simulink model "NE_Red_Rooster_Delta_B_28may"  (R2019b)
settings: Solver=FixedStepAuto  StartTime=0.0  StopTime=inf  FixedStep=0.0005  RelTol=1e-3
PreLoadFcn:
  | waijung.modelPreload; % Required for working with Waijung Blockset. Do not remove.
undefined symbols (not defined in the file): ARM, DiscIntNeverNeededParam, HSEOSC, Link, LQFP100, MDK, ST, STM32F407VG
libraries: simulink x30, stm32f4_i2c_lib x22, stm32f4_io_lib x6, stm32f4_reset_lib x1, stm32f4_device_config_lib x1
(part 2 of 5)

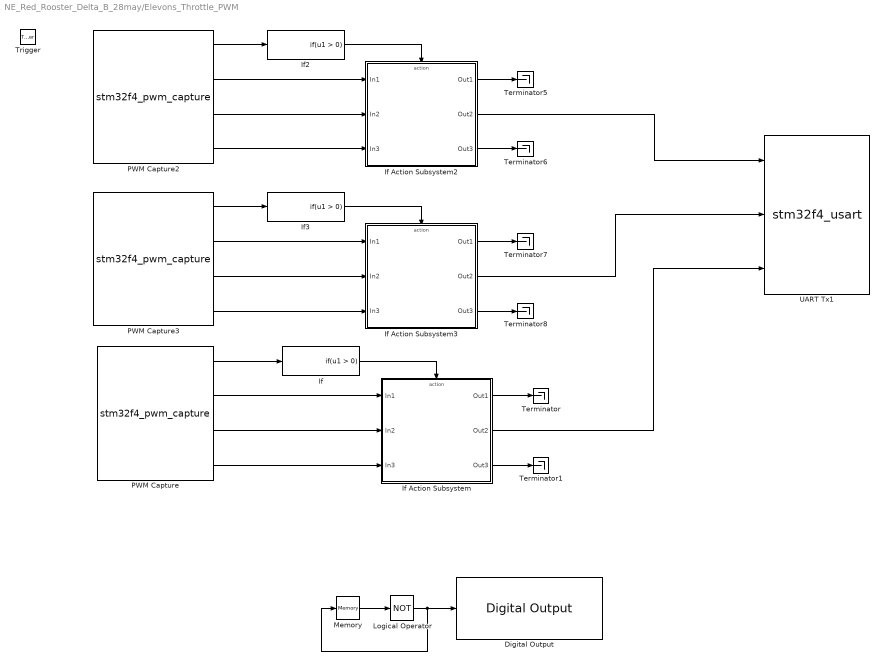
== system NE_Red_Rooster_Delta_B_28may/Elevons_Throttle_PWM ==
  Trigger : TriggerPort  VariantControl=Variant
  Digital Output : stm32f4_io_lib/Digital Output  use_bitband=on  port=D  speed=100  porttype=Push Pull  porttypestr=PP  use_pin0=off  use_pin1=off  use_pin2=off  use_pin3=off  use_pin4=off  use_pin5=off  use_pin6=off  use_pin7=off  use_pin8=off  use_pin9=off  use_pin10=off  use_pin11=off  use_pin12=on  use_pin13=off  use_pin14=off  use_pin15=off  pinstr=GPIO_Pin_12  usedpinarray="[0  0  0  0  0  0  0  0  0  0  0  0  1  0  0  0]"  bitbandingstr="#define Elevons_Throttle_PWMDigitalOutput_D12 Peripheral_BB(GPIOD->ODR, 12)  /* Output pin */"  sampletime=-1  sampletimestr=-1  blockid=Elevons_Throttle_PWMDigitalOutput  enablecustomportlabel=off  globalinit=off  cinputportlabel=In1, In2  coutputportlabel=0
  If : If  ShowElse=off
  If Action Subsystem : Subsystem  TreatAsAtomicUnit=on
  If Action Subsystem2 : Subsystem  TreatAsAtomicUnit=on
  If Action Subsystem3 : Subsystem  TreatAsAtomicUnit=on
  If2 : If  ShowElse=off
  If3 : If  ShowElse=off
  Logical Operator : Logic  Operator=NOT  AllPortsSameDT=off  OutDataTypeStr=boolean
  Memory : Memory  InheritSampleTime=on
  PWM Capture : S-Function  FunctionName=stm32f4_pwm_capture  Parameters=conf,inputporttype,inputportwidth,outputporttype,outputportwidth,optionstring,sampletime,blockid  SFunctionDeploymentMode=off  EnableBusSupport=off  mask(stm32f4_pwm_capture){conf=Capture, timer=8, lasttimer=8, pin=C6, pintype=Pull Up, edge=Rising, datatype=single, portpinstr=0, sampletime=-1, blockid=Elevons_Throttle_PWMPWMCapture, inputporttype=[], inputportwidth=[], inputportlabel={}, outputporttype=[3 1 1 1], outputportwidth=[], outputportlabel={'READY','+Width (sec)','+Duty (%)','Frequency (Hz)'}, compat=0, optionstring=["8","2","C","6","1","16","Rising","UP","float"]}
      mask prompts: conf "Configuration"; lasttimer "Last Timer"; pin "Capture Pin"; pintype "Capture Pin Type (Pull-Up/Pull-Down)"; edge "Capture Edge"; datatype "Output data type"; portpinstr "Port Pin String"; sampletime "Sample time (sec)"; blockid "Block ID"; inputporttype "Input Port Type"; inputportwidth "Input Port Width"; inputportlabel "Input Port Label"; outputporttype "Output Port Type"; outputportwidth "Output Port Width"; outputportlabel "Output port label"; compat "Compatibility (Reserved for future use)"; optionstring "String(s) to be passed to TLC"
      mask help:
      | Capture Edge:
      |  Rising - PWM period start from rising edge of pulse N to rising edge of pulse N+1
      |  Falling - PWM period start from falling edge of pulse N to falling edge of pulse N+1
      | Capture data type:
      |  Capture data type, selectable to double or single.
      |
      | Output:
      |  READY - indicate the status of capture, a non-zero value indicate data is ready.
      |  +Width - positive pulse width, in unit of second.
      |  +Duty - positive duty cycle, 0 to 100%
      |  Frequency - signal frequency in unit of Hz
      |
      | Note: caprure period should not longer than 1 second (Maximum limit is 3 seconds)
      mask init:
      | stm32f4_pwm_capture_callback('init');
      mask Help: web(fullfile(waijungdocroot,'stm32f4_pwm_capture.htm'), '-browser')
      mask TypeOptions conf: Capture
      mask Callback conf: stm32f4_pwm_capture_callback('conf');
      mask TypeOptions timer: 1 | 2 | 3 | 4 | 5 | 8
      mask Callback timer: stm32f4_pwm_capture_callback('timer');
      mask TypeOptions pin: Not used | C6 | C7 | C8 | C9
      mask TypeOptions pintype: None | Pull Up | Pull Down
      mask TypeOptions edge: Rising | Falling
      mask TypeOptions datatype: double | single
      mask Callback sampletime: stm32f4_pwm_capture_callback('sampletime');
      mask Callback blockid: stm32f4_pwm_capture_callback('blockid');
      mask Display: text(0.05, 0.5, 'Timer: 8 (16 bit)\nInput Pin: C6\nEdge: Rising\nTs (sec): -1','ver','middle','hor','left'); port_label('output', 1,'READY'); port_label('output', 2,'+Width (sec)'); port_label('output', 3,'+Duty (%)'); port_label('output', 4,'Frequency (Hz)');
  PWM Capture2 : S-Function  FunctionName=stm32f4_pwm_capture  Parameters=conf,inputporttype,inputportwidth,outputporttype,outputportwidth,optionstring,sampletime,blockid  SFunctionDeploymentMode=off  EnableBusSupport=off  mask(stm32f4_pwm_capture){conf=Capture, timer=1, lasttimer=1, pin=E9, pintype=Pull Up, edge=Rising, datatype=single, portpinstr=0, sampletime=-1, blockid=Elevons_Throttle_PWMPWMCapture2, inputporttype=[], inputportwidth=[], inputportlabel={}, outputporttype=[3 1 1 1], outputportwidth=[], outputportlabel={'READY','+Width (sec)','+Duty (%)','Frequency (Hz)'}, compat=0, optionstring=["1","2","E","9","1","16","Rising","UP","float"]}
      mask prompts: conf "Configuration"; lasttimer "Last Timer"; pin "Capture Pin"; pintype "Capture Pin Type (Pull-Up/Pull-Down)"; edge "Capture Edge"; datatype "Output data type"; portpinstr "Port Pin String"; sampletime "Sample time (sec)"; blockid "Block ID"; inputporttype "Input Port Type"; inputportwidth "Input Port Width"; inputportlabel "Input Port Label"; outputporttype "Output Port Type"; outputportwidth "Output Port Width"; outputportlabel "Output port label"; compat "Compatibility (Reserved for future use)"; optionstring "String(s) to be passed to TLC"
      mask help:
      | Capture Edge:
      |  Rising - PWM period start from rising edge of pulse N to rising edge of pulse N+1
      |  Falling - PWM period start from falling edge of pulse N to falling edge of pulse N+1
      | Capture data type:
      |  Capture data type, selectable to double or single.
      |
      | Output:
      |  READY - indicate the status of capture, a non-zero value indicate data is ready.
      |  +Width - positive pulse width, in unit of second.
      |  +Duty - positive duty cycle, 0 to 100%
      |  Frequency - signal frequency in unit of Hz
      |
      | Note: caprure period should not longer than 1 second (Maximum limit is 3 seconds)
      mask init:
      | stm32f4_pwm_capture_callback('init');
      mask Help: web(fullfile(waijungdocroot,'stm32f4_pwm_capture.htm'), '-browser')
      mask TypeOptions conf: Capture
      mask Callback conf: stm32f4_pwm_capture_callback('conf');
      mask TypeOptions timer: 1 | 2 | 3 | 4 | 5 | 8
      mask Callback timer: stm32f4_pwm_capture_callback('timer');
      mask TypeOptions pin: Not used | A8 | E9 | A9 | E11 | A10 | E13 | A11 | E14
      mask TypeOptions pintype: None | Pull Up | Pull Down
      mask TypeOptions edge: Rising | Falling
      mask TypeOptions datatype: double | single
      mask Callback sampletime: stm32f4_pwm_capture_callback('sampletime');
      mask Callback blockid: stm32f4_pwm_capture_callback('blockid');
      mask Display: text(0.05, 0.5, 'Timer: 1 (16 bit)\nInput Pin: E9\nEdge: Rising\nTs (sec): -1','ver','middle','hor','left'); port_label('output', 1,'READY'); port_label('output', 2,'+Width (sec)'); port_label('output', 3,'+Duty (%)'); port_label('output', 4,'Frequency (Hz)');
  PWM Capture3 : S-Function  FunctionName=stm32f4_pwm_capture  Parameters=conf,inputporttype,inputportwidth,outputporttype,outputportwidth,optionstring,sampletime,blockid  SFunctionDeploymentMode=off  EnableBusSupport=off  mask(stm32f4_pwm_capture){conf=Capture, timer=3, lasttimer=3, pin=C7, pintype=Pull Up, edge=Rising, datatype=single, portpinstr=0, sampletime=-1, blockid=Elevons_Throttle_PWMPWMCapture3, inputporttype=[], inputportwidth=[], inputportlabel={}, outputporttype=[3 1 1 1], outputportwidth=[], outputportlabel={'READY','+Width (sec)','+Duty (%)','Frequency (Hz)'}, compat=0, optionstring=["3","1","C","7","2","16","Rising","UP","float"]}
      mask prompts: conf "Configuration"; lasttimer "Last Timer"; pin "Capture Pin"; pintype "Capture Pin Type (Pull-Up/Pull-Down)"; edge "Capture Edge"; datatype "Output data type"; portpinstr "Port Pin String"; sampletime "Sample time (sec)"; blockid "Block ID"; inputporttype "Input Port Type"; inputportwidth "Input Port Width"; inputportlabel "Input Port Label"; outputporttype "Output Port Type"; outputportwidth "Output Port Width"; outputportlabel "Output port label"; compat "Compatibility (Reserved for future use)"; optionstring "String(s) to be passed to TLC"
      mask help:
      | Capture Edge:
      |  Rising - PWM period start from rising edge of pulse N to rising edge of pulse N+1
      |  Falling - PWM period start from falling edge of pulse N to falling edge of pulse N+1
      | Capture data type:
      |  Capture data type, selectable to double or single.
      |
      | Output:
      |  READY - indicate the status of capture, a non-zero value indicate data is ready.
      |  +Width - positive pulse width, in unit of second.
      |  +Duty - positive duty cycle, 0 to 100%
      |  Frequency - signal frequency in unit of Hz
      |
      | Note: caprure period should not longer than 1 second (Maximum limit is 3 seconds)
      mask init:
      | stm32f4_pwm_capture_callback('init');
      mask Help: web(fullfile(waijungdocroot,'stm32f4_pwm_capture.htm'), '-browser')
      mask TypeOptions conf: Capture
      mask Callback conf: stm32f4_pwm_capture_callback('conf');
      mask TypeOptions timer: 1 | 2 | 3 | 4 | 5 | 8
      mask Callback timer: stm32f4_pwm_capture_callback('timer');
      mask TypeOptions pin: Not used | A6 | B4 | C6 | A7 | B5 | C7 | B0 | C8 | B1 | C9
      mask TypeOptions pintype: None | Pull Up | Pull Down
      mask TypeOptions edge: Rising | Falling
      mask TypeOptions datatype: double | single
      mask Callback sampletime: stm32f4_pwm_capture_callback('sampletime');
      mask Callback blockid: stm32f4_pwm_capture_callback('blockid');
      mask Display: text(0.05, 0.5, 'Timer: 3 (16 bit)\nInput Pin: C7\nEdge: Rising\nTs (sec): -1','ver','middle','hor','left'); port_label('output', 1,'READY'); port_label('output', 2,'+Width (sec)'); port_label('output', 3,'+Duty (%)'); port_label('output', 4,'Frequency (Hz)');
  Terminator{,1,5..8} (6 alike) : Terminator
  UART Tx1 : S-Function  Priority=1  FunctionName=stm32f4_usart  Parameters=configuration,uartmodule,transfer,baudrate,inputtype,outputtype,confstr,binheaderarray,binterminatorarray,asciiheader,asciiterminator,bindatalength,packetmode,varname,sampletime,sampletimestr,blockid  SFunctionDeploymentMode=off  EnableBusSupport=off  mask(stm32f4_usart){configuration=Tx, uartmodule=2, baudrate=115200, databits=8, parity=No, stopbit=1, remaptxpin=Not used, remaprxpin=Not used, flowcontrol=None, remapctspin=Not used, remaprtspin=Not used, advanceoptions=off, rxbuffersize=512, txbuffersize=512, transfer=Blocking, packetmode=Binary, binheader='45', binterminator='2E', porttype_double=0, porttype_single=3, porttype_int8=0, porttype_uint8=0, porttype_int16=0, porttype_uint16=0, porttype_int32=0, porttype_uint32=0, asciiformat='%f, %f', rx_asciiterminator=CRLF (0x0D 0x0A - "\r\n"), tx_asciiterminator=CRLF (0x0D 0x0A - "\r\n"), storagename=<empty>, varname=, inputtype=[3  1 1 1], outputtype=[0], binheaderarray=[1 69], binterminatorarray=[1 46], bindatalength=12, asciiheader='%f, %f\r\n', asciiterminator=[2 13 10], sampletime=-1, sampletimestr=-1, blockid=Elevons_Throttle_PWMUARTTx1, confstr=[ "dummy", "0", "*", "*", "0", "*", "*", "0", "*", "*", "0", "*", "*", "1", "4", "6", "1", "4", "5", "512", "512", "1", "2", "115200", "8", "No", "1", "None", "USART2"], lastmodule=1}
      mask prompts: uartmodule "UART Module"; baudrate "Baud rate (bps)"; databits "Data bits"; stopbit "Stop bit"; remaptxpin "Tx Pin"; remaprxpin "Rx Pin"; flowcontrol "Hardware flow control"; remapctspin "HW Flow control, CTS Pin"; remaprtspin "HW Flow control, RTS Pin"; advanceoptions "Advance options"; rxbuffersize "Rx buffer size (bytes)"; txbuffersize "Tx buffer size (bytes)"; packetmode "Packet mode"; binheader "Binary header (example: '7E 7E')"; binterminator "Binary terminator (example: '03 03')"; porttype_double "Number of data port, type DOUBLE"; porttype_single "Number of data port, type SINGLE"; porttype_int8 "Number of data port, type INT8"; porttype_uint8 "Number of data port, type UINT8"; porttype_int16 "Number of data port, type INT16"; porttype_uint16 "Number of data port, type UINT16"; porttype_int32 "Number of data port, type INT32"; porttype_uint32 "Number of data port, type UINT32"; asciiformat "Ascii format"; rx_asciiterminator "End of packet"; tx_asciiterminator "End of packet"; storagename "Buffer"; varname "Var name"; inputtype "Input data type"; outputtype "Output data type"; binheaderarray "Binary header"; binterminatorarray "Binary terminator"; bindatalength "Binary data length"; asciiheader "Ascii header (printf format)"; asciiterminator "Ascii terminator"; sampletime "Sample time (sec)"; sampletimestr "Compiled sample time (sec) in string"; confstr "Configuration string"; lastmodule "Last module selected"
      mask help:
      | Data type for Ascii format
      | %u, %i, %d, %o, %x: uint32
      | %e, %g, %f: single
      | %c: int8
      mask init:
      | stm32f4_usart_callback('init');
      mask Help: web(fullfile(waijungdocroot,'stm32f4_usart_tx.htm'), '-browser')
      mask TypeOptions configuration: Setup | Tx | Rx
      mask Callback configuration: stm32f4_usart_callback('configuration');
      mask TypeOptions uartmodule: 1 | 2 | 3 | 4 | 5 | 6
      mask Callback uartmodule: stm32f4_usart_callback('uartmodule');
      mask Callback baudrate: stm32f4_usart_callback('baudrate');
      mask TypeOptions databits: 8
      mask TypeOptions parity: No | Odd | Even
      mask TypeOptions stopbit: 0.5 | 1 | 1.5 | 2
      mask TypeOptions remaptxpin: Not used | A9 | B6
      mask TypeOptions remaprxpin: Not used | A10 | B7
      mask TypeOptions flowcontrol: None | RTS | CTS | RTS/CTS
      mask Callback flowcontrol: stm32f4_usart_callback('flowcontrol');
      mask TypeOptions remapctspin: Not used | A11
      mask TypeOptions remaprtspin: Not used | A12
      mask Callback advanceoptions: stm32f4_usart_callback('advanceoptions');
      mask TypeOptions rxbuffersize: 16 | 32 | 64 | 128 | 256 | 512 | 1024 | 2048
      mask TypeOptions txbuffersize: 16 | 32 | 64 | 128 | 256 | 512 | 1024 | 2048
      mask TypeOptions transfer: Blocking | Non-Blocking
      mask Callback transfer: stm32f4_usart_callback('transfer');
      mask TypeOptions packetmode: Ascii | Binary | Binary Vector | String Buffer | Raw Buffer
      mask Callback packetmode: stm32f4_usart_callback('packetmode');
      mask Callback binheader: stm32f4_usart_callback('binheader');
      mask Callback binterminator: stm32f4_usart_callback('binterminator');
      mask Callback porttype_double: stm32f4_usart_callback('porttype');
      mask Callback porttype_single: stm32f4_usart_callback('porttype');
      mask Callback porttype_int8: stm32f4_usart_callback('porttype');
      mask Callback porttype_uint8: stm32f4_usart_callback('porttype');
      mask Callback porttype_int16: stm32f4_usart_callback('porttype');
      mask Callback porttype_uint16: stm32f4_usart_callback('porttype');
      mask Callback porttype_int32: stm32f4_usart_callback('porttype');
      mask Callback porttype_uint32: stm32f4_usart_callback('porttype');
      mask Callback asciiformat: stm32f4_usart_callback('asciiformat');
      mask TypeOptions rx_asciiterminator: CR (0x0D - "\r") | LF (0x0A - "\n") | CRLF (0x0D 0x0A - "\r\n")
      mask Callback rx_asciiterminator: stm32f4_usart_callback('rx_asciiterminator');
      mask TypeOptions tx_asciiterminator: CR (0x0D - "\r") | LF (0x0A - "\n") | CRLF (0x0D 0x0A - "\r\n") | None
      mask Callback tx_asciiterminator: stm32f4_usart_callback('tx_asciiterminator');
      mask TypeOptions storagename: <empty>
      mask Callback storagename: stm32f4_usart_callback('storagename');
      mask Callback varname: stm32f4_usart_callback('varname');
      mask Callback sampletime: stm32f4_usart_callback('sampletime');
      mask Callback sampletimestr: stm32f4_usart_callback('sampletimestr');
      mask Callback blockid: stm32f4_usart_callback('blockid');
      mask Display: text(0.95, 0.5, 'Module: USART2_Tx\nPacket: Binary\nTransfer: Blocking\nTs (sec): -1','ver','middle','hor','right'); port_label('input', 1,'single'); port_label('input', 2,'single'); port_label('input', 3,'single');
  wires:
  If/1 -> If Action Subsystem/Action
  PWM Capture/1 -> If/1
  PWM Capture/2 -> If Action Subsystem/1(In1)
  PWM Capture/3 -> If Action Subsystem/2(In2)
  PWM Capture/4 -> If Action Subsystem/3(In3)
  If Action Subsystem/1(Out1) -> Terminator/1
  If Action Subsystem/3(Out3) -> Terminator1/1
  If Action Subsystem2/2(Out2) -> UART Tx1/1
  If Action Subsystem3/2(Out2) -> UART Tx1/2
  If Action Subsystem/2(Out2) -> UART Tx1/3
  Memory/1 -> Logical Operator/1
  Logical Operator/1 -> Digital Output/1, Memory/1
  If3/1 -> If Action Subsystem3/Action
  PWM Capture3/2 -> If Action Subsystem3/1(In1)
  PWM Capture3/3 -> If Action Subsystem3/2(In2)
  PWM Capture3/4 -> If Action Subsystem3/3(In3)
  If Action Subsystem3/1(Out1) -> Terminator7/1
  If Action Subsystem3/3(Out3) -> Terminator8/1
  PWM Capture3/1 -> If3/1
  If2/1 -> If Action Subsystem2/Action
  PWM Capture2/1 -> If2/1
  PWM Capture2/2 -> If Action Subsystem2/1(In1)
  PWM Capture2/3 -> If Action Subsystem2/2(In2)
  PWM Capture2/4 -> If Action Subsystem2/3(In3)
  If Action Subsystem2/1(Out1) -> Terminator5/1
  If Action Subsystem2/3(Out3) -> Terminator6/1

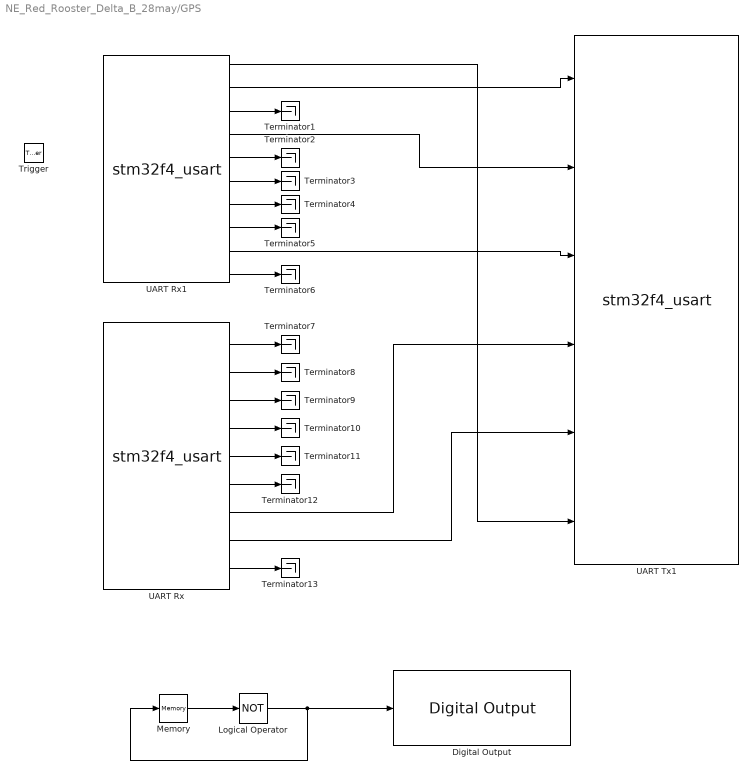
== system NE_Red_Rooster_Delta_B_28may/GPS ==
  Trigger : TriggerPort  VariantControl=Variant
  Digital Output : stm32f4_io_lib/Digital Output  use_bitband=on  port=D  speed=100  porttype=Push Pull  porttypestr=PP  use_pin0=off  use_pin1=off  use_pin2=off  use_pin3=off  use_pin4=off  use_pin5=off  use_pin6=off  use_pin7=off  use_pin8=off  use_pin9=off  use_pin10=off  use_pin11=off  use_pin12=off  use_pin13=off  use_pin14=off  use_pin15=on  pinstr=GPIO_Pin_15  usedpinarray="[0  0  0  0  0  0  0  0  0  0  0  0  0  0  0  1]"  bitbandingstr="#define GPSDigitalOutput_D15 Peripheral_BB(GPIOD->ODR, 15)  /* Output pin */"  sampletime=-1  sampletimestr=-1  blockid=GPSDigitalOutput  enablecustomportlabel=off  globalinit=off  cinputportlabel=In1, In2  coutputportlabel=0
  Logical Operator : Logic  Operator=NOT  AllPortsSameDT=off  OutDataTypeStr=boolean
  Memory : Memory  InheritSampleTime=on
  Terminator{1..13} (13 alike) : Terminator
  UART Rx : S-Function  Priority=1  FunctionName=stm32f4_usart  Parameters=configuration,uartmodule,transfer,baudrate,inputtype,outputtype,confstr,binheaderarray,binterminatorarray,asciiheader,asciiterminator,bindatalength,packetmode,varname,sampletime,sampletimestr,blockid  SFunctionDeploymentMode=off  EnableBusSupport=off  mask(stm32f4_usart){configuration=Rx, uartmodule=3, baudrate=115200, databits=8, parity=No, stopbit=1, remaptxpin=Not used, remaprxpin=Not used, flowcontrol=None, remapctspin=Not used, remaprtspin=Not used, advanceoptions=off, rxbuffersize=512, txbuffersize=512, transfer=Blocking, packetmode=Ascii, binheader='7E 7E', binterminator='03 03', porttype_double=1, porttype_single=0, porttype_int8=1, porttype_uint8=0, porttype_int16=0, porttype_uint16=0, porttype_int32=0, porttype_uint32=0, asciiformat='$GPRMC,%f,%c,%f,%c,%f,%c,%f,%f,%u,,,', rx_asciiterminator=CRLF (0x0D 0x0A - "\r\n"), tx_asciiterminator=LF (0x0A - "\n"), storagename=D0, varname=, inputtype=[0], outputtype=[9  1 2 1 2 1 2 1 1 7], binheaderarray=[0], binterminatorarray=[0], bindatalength=0, asciiheader='$GPRMC,%f,%c,%f,%c,%f,%c,%f,%f,%u,,,\r\n', asciiterminator=[2 13 10], sampletime=-1, sampletimestr=-1, blockid=GPSUARTRx, confstr=[ "dummy", "0", "*", "*", "0", "*", "*", "0", "*", "*", "0", "*", "*", "1", "4", "3", "1", "4", "1", "512", "512", "1", "3", "115200", "8", "No", "1", "None", "USART3"], lastmodule=1}
      mask prompts: uartmodule "UART Module"; baudrate "Baud rate (bps)"; databits "Data bits"; stopbit "Stop bit"; remaptxpin "Tx Pin"; remaprxpin "Rx Pin"; flowcontrol "Hardware flow control"; remapctspin "HW Flow control, CTS Pin"; remaprtspin "HW Flow control, RTS Pin"; advanceoptions "Advance options"; rxbuffersize "Rx buffer size (bytes)"; txbuffersize "Tx buffer size (bytes)"; packetmode "Packet mode"; binheader "Binary header (example: '7E 7E')"; binterminator "Binary terminator (example: '03 03')"; porttype_double "Number of data port, type DOUBLE"; porttype_single "Number of data port, type SINGLE"; porttype_int8 "Number of data port, type INT8"; porttype_uint8 "Number of data port, type UINT8"; porttype_int16 "Number of data port, type INT16"; porttype_uint16 "Number of data port, type UINT16"; porttype_int32 "Number of data port, type INT32"; porttype_uint32 "Number of data port, type UINT32"; asciiformat "Ascii format"; rx_asciiterminator "End of packet"; tx_asciiterminator "End of packet"; storagename "Buffer"; varname "Var name"; inputtype "Input data type"; outputtype "Output data type"; binheaderarray "Binary header"; binterminatorarray "Binary terminator"; bindatalength "Binary data length"; asciiheader "Ascii header (printf format)"; asciiterminator "Ascii terminator"; sampletime "Sample time (sec)"; sampletimestr "Compiled sample time (sec) in string"; confstr "Configuration string"; lastmodule "Last module selected"
      mask init:
      | stm32f4_usart_callback('init');
      mask Help: web(fullfile(waijungdocroot,'stm32f4_usart_rx.htm'), '-browser')
      mask TypeOptions configuration: Setup | Tx | Rx
      mask Callback configuration: stm32f4_usart_callback('configuration');
      mask TypeOptions uartmodule: 1 | 2 | 3 | 4 | 5 | 6
      mask Callback uartmodule: stm32f4_usart_callback('uartmodule');
      mask Callback baudrate: stm32f4_usart_callback('baudrate');
      mask TypeOptions databits: 8
      mask TypeOptions parity: No | Odd | Even
      mask TypeOptions stopbit: 0.5 | 1 | 1.5 | 2
      mask TypeOptions remaptxpin: Not used | A9 | B6
      mask TypeOptions remaprxpin: Not used | A10 | B7
      mask TypeOptions flowcontrol: None | RTS | CTS | RTS/CTS
      mask Callback flowcontrol: stm32f4_usart_callback('flowcontrol');
      mask TypeOptions remapctspin: Not used | A11
      mask TypeOptions remaprtspin: Not used | A12
      mask Callback advanceoptions: stm32f4_usart_callback('advanceoptions');
      mask TypeOptions rxbuffersize: 16 | 32 | 64 | 128 | 256 | 512 | 1024 | 2048
      mask TypeOptions txbuffersize: 16 | 32 | 64 | 128 | 256 | 512 | 1024 | 2048
      mask TypeOptions transfer: Blocking | Non-Blocking
      mask Callback transfer: stm32f4_usart_callback('transfer');
      mask TypeOptions packetmode: Ascii | Binary | String Buffer
      mask Callback packetmode: stm32f4_usart_callback('packetmode');
      mask Callback binheader: stm32f4_usart_callback('binheader');
      mask Callback binterminator: stm32f4_usart_callback('binterminator');
      mask Callback porttype_double: stm32f4_usart_callback('porttype');
      mask Callback porttype_single: stm32f4_usart_callback('porttype');
      mask Callback porttype_int8: stm32f4_usart_callback('porttype');
      mask Callback porttype_uint8: stm32f4_usart_callback('porttype');
      mask Callback porttype_int16: stm32f4_usart_callback('porttype');
      mask Callback porttype_uint16: stm32f4_usart_callback('porttype');
      mask Callback porttype_int32: stm32f4_usart_callback('porttype');
      mask Callback porttype_uint32: stm32f4_usart_callback('porttype');
      mask Callback asciiformat: stm32f4_usart_callback('asciiformat');
      mask TypeOptions rx_asciiterminator: CR (0x0D - "\r") | LF (0x0A - "\n") | CRLF (0x0D 0x0A - "\r\n")
      mask Callback rx_asciiterminator: stm32f4_usart_callback('rx_asciiterminator');
      mask TypeOptions tx_asciiterminator: CR (0x0D - "\r") | LF (0x0A - "\n") | CRLF (0x0D 0x0A - "\r\n") | None
      mask Callback tx_asciiterminator: stm32f4_usart_callback('tx_asciiterminator');
      mask TypeOptions storagename: D0
      mask Callback storagename: stm32f4_usart_callback('storagename');
      mask Callback varname: stm32f4_usart_callback('varname');
      mask Callback sampletime: stm32f4_usart_callback('sampletime');
      mask Callback sampletimestr: stm32f4_usart_callback('sampletimestr');
      mask Callback blockid: stm32f4_usart_callback('blockid');
      mask Display: text(0.05, 0.5, 'Module: USART3_Rx\nPacket: Ascii\nTransfer: Blocking\nTs (sec): -1','ver','middle','hor','left'); port_label('output', 1,'single'); port_label('output', 2,'int8'); port_label('output', 3,'single'); port_label('output', 4,'int8'); port_label('output', 5,'single'); port_label('output', 6,'int8'); port_label('output', 7,'single'); port_label('output', 8,'single'); port_label('output', 9,'uint32');
  UART Rx1 : S-Function  Priority=1  FunctionName=stm32f4_usart  Parameters=configuration,uartmodule,transfer,baudrate,inputtype,outputtype,confstr,binheaderarray,binterminatorarray,asciiheader,asciiterminator,bindatalength,packetmode,varname,sampletime,sampletimestr,blockid  SFunctionDeploymentMode=off  EnableBusSupport=off  mask(stm32f4_usart){configuration=Rx, uartmodule=3, baudrate=115200, databits=8, parity=No, stopbit=1, remaptxpin=Not used, remaprxpin=Not used, flowcontrol=None, remapctspin=Not used, remaprtspin=Not used, advanceoptions=off, rxbuffersize=512, txbuffersize=512, transfer=Blocking, packetmode=Ascii, binheader='7E 7E', binterminator='03 03', porttype_double=1, porttype_single=0, porttype_int8=1, porttype_uint8=0, porttype_int16=0, porttype_uint16=0, porttype_int32=0, porttype_uint32=0, asciiformat='$GPGGA,%f,%f,%c,%f,%c,%c,%c,%f,%f,%c,,,,', rx_asciiterminator=CRLF (0x0D 0x0A - "\r\n"), tx_asciiterminator=LF (0x0A - "\n"), storagename=D0, varname=, inputtype=[0], outputtype=[10  1 1 2 1 2 2 2 1 1 2], binheaderarray=[0], binterminatorarray=[0], bindatalength=0, asciiheader='$GPGGA,%f,%f,%c,%f,%c,%c,%c,%f,%f,%c,,,,\r\n', asciiterminator=[2 13 10], sampletime=-1, sampletimestr=-1, blockid=GPSUARTRx1, confstr=[ "dummy", "0", "*", "*", "0", "*", "*", "0", "*", "*", "0", "*", "*", "1", "4", "3", "1", "4", "1", "512", "512", "1", "3", "115200", "8", "No", "1", "None", "USART3"], lastmodule=1}
      mask prompts: uartmodule "UART Module"; baudrate "Baud rate (bps)"; databits "Data bits"; stopbit "Stop bit"; remaptxpin "Tx Pin"; remaprxpin "Rx Pin"; flowcontrol "Hardware flow control"; remapctspin "HW Flow control, CTS Pin"; remaprtspin "HW Flow control, RTS Pin"; advanceoptions "Advance options"; rxbuffersize "Rx buffer size (bytes)"; txbuffersize "Tx buffer size (bytes)"; packetmode "Packet mode"; binheader "Binary header (example: '7E 7E')"; binterminator "Binary terminator (example: '03 03')"; porttype_double "Number of data port, type DOUBLE"; porttype_single "Number of data port, type SINGLE"; porttype_int8 "Number of data port, type INT8"; porttype_uint8 "Number of data port, type UINT8"; porttype_int16 "Number of data port, type INT16"; porttype_uint16 "Number of data port, type UINT16"; porttype_int32 "Number of data port, type INT32"; porttype_uint32 "Number of data port, type UINT32"; asciiformat "Ascii format"; rx_asciiterminator "End of packet"; tx_asciiterminator "End of packet"; storagename "Buffer"; varname "Var name"; inputtype "Input data type"; outputtype "Output data type"; binheaderarray "Binary header"; binterminatorarray "Binary terminator"; bindatalength "Binary data length"; asciiheader "Ascii header (printf format)"; asciiterminator "Ascii terminator"; sampletime "Sample time (sec)"; sampletimestr "Compiled sample time (sec) in string"; confstr "Configuration string"; lastmodule "Last module selected"
      mask init:
      | stm32f4_usart_callback('init');
      mask Help: web(fullfile(waijungdocroot,'stm32f4_usart_rx.htm'), '-browser')
      mask TypeOptions configuration: Setup | Tx | Rx
      mask Callback configuration: stm32f4_usart_callback('configuration');
      mask TypeOptions uartmodule: 1 | 2 | 3 | 4 | 5 | 6
      mask Callback uartmodule: stm32f4_usart_callback('uartmodule');
      mask Callback baudrate: stm32f4_usart_callback('baudrate');
      mask TypeOptions databits: 8
      mask TypeOptions parity: No | Odd | Even
      mask TypeOptions stopbit: 0.5 | 1 | 1.5 | 2
      mask TypeOptions remaptxpin: Not used | A9 | B6
      mask TypeOptions remaprxpin: Not used | A10 | B7
      mask TypeOptions flowcontrol: None | RTS | CTS | RTS/CTS
      mask Callback flowcontrol: stm32f4_usart_callback('flowcontrol');
      mask TypeOptions remapctspin: Not used | A11
      mask TypeOptions remaprtspin: Not used | A12
      mask Callback advanceoptions: stm32f4_usart_callback('advanceoptions');
      mask TypeOptions rxbuffersize: 16 | 32 | 64 | 128 | 256 | 512 | 1024 | 2048
      mask TypeOptions txbuffersize: 16 | 32 | 64 | 128 | 256 | 512 | 1024 | 2048
      mask TypeOptions transfer: Blocking | Non-Blocking
      mask Callback transfer: stm32f4_usart_callback('transfer');
      mask TypeOptions packetmode: Ascii | Binary | String Buffer
      mask Callback packetmode: stm32f4_usart_callback('packetmode');
      mask Callback binheader: stm32f4_usart_callback('binheader');
      mask Callback binterminator: stm32f4_usart_callback('binterminator');
      mask Callback porttype_double: stm32f4_usart_callback('porttype');
      mask Callback porttype_single: stm32f4_usart_callback('porttype');
      mask Callback porttype_int8: stm32f4_usart_callback('porttype');
      mask Callback porttype_uint8: stm32f4_usart_callback('porttype');
      mask Callback porttype_int16: stm32f4_usart_callback('porttype');
      mask Callback porttype_uint16: stm32f4_usart_callback('porttype');
      mask Callback porttype_int32: stm32f4_usart_callback('porttype');
      mask Callback porttype_uint32: stm32f4_usart_callback('porttype');
      mask Callback asciiformat: stm32f4_usart_callback('asciiformat');
      mask TypeOptions rx_asciiterminator: CR (0x0D - "\r") | LF (0x0A - "\n") | CRLF (0x0D 0x0A - "\r\n")
      mask Callback rx_asciiterminator: stm32f4_usart_callback('rx_asciiterminator');
      mask TypeOptions tx_asciiterminator: CR (0x0D - "\r") | LF (0x0A - "\n") | CRLF (0x0D 0x0A - "\r\n") | None
      mask Callback tx_asciiterminator: stm32f4_usart_callback('tx_asciiterminator');
      mask TypeOptions storagename: D0
      mask Callback storagename: stm32f4_usart_callback('storagename');
      mask Callback varname: stm32f4_usart_callback('varname');
      mask Callback sampletime: stm32f4_usart_callback('sampletime');
      mask Callback sampletimestr: stm32f4_usart_callback('sampletimestr');
      mask Callback blockid: stm32f4_usart_callback('blockid');
      mask Display: text(0.05, 0.5, 'Module: USART3_Rx\nPacket: Ascii\nTransfer: Blocking\nTs (sec): -1','ver','middle','hor','left'); port_label('output', 1,'single'); port_label('output', 2,'single'); port_label('output', 3,'int8'); port_label('output', 4,'single'); port_label('output', 5,'int8'); port_label('output', 6,'int8'); port_label('output', 7,'int8'); port_label('output', 8,'single'); port_label('output', 9,'single'); port_label('output', 10,'int8');
  UART Tx1 : S-Function  Priority=1  FunctionName=stm32f4_usart  Parameters=configuration,uartmodule,transfer,baudrate,inputtype,outputtype,confstr,binheaderarray,binterminatorarray,asciiheader,asciiterminator,bindatalength,packetmode,varname,sampletime,sampletimestr,blockid  SFunctionDeploymentMode=off  EnableBusSupport=off  mask(stm32f4_usart){configuration=Tx, uartmodule=2, baudrate=115200, databits=8, parity=No, stopbit=1, remaptxpin=Not used, remaprxpin=Not used, flowcontrol=None, remapctspin=Not used, remaprtspin=Not used, advanceoptions=off, rxbuffersize=512, txbuffersize=512, transfer=Blocking, packetmode=Binary, binheader='53', binterminator='2E', porttype_double=0, porttype_single=6, porttype_int8=0, porttype_uint8=0, porttype_int16=0, porttype_uint16=0, porttype_int32=0, porttype_uint32=0, asciiformat='Alt=%f', rx_asciiterminator=CRLF (0x0D 0x0A - "\r\n"), tx_asciiterminator=CRLF (0x0D 0x0A - "\r\n"), storagename=<empty>, varname=, inputtype=[6  1 1 1 1 1 1], outputtype=[0], binheaderarray=[1 83], binterminatorarray=[1 46], bindatalength=24, asciiheader='Alt=%f\r\n', asciiterminator=[2 13 10], sampletime=-1, sampletimestr=-1, blockid=GPSUARTTx1, confstr=[ "dummy", "0", "*", "*", "0", "*", "*", "0", "*", "*", "0", "*", "*", "1", "4", "6", "1", "4", "5", "512", "512", "1", "2", "115200", "8", "No", "1", "None", "USART2"], lastmodule=1}
      mask prompts: uartmodule "UART Module"; baudrate "Baud rate (bps)"; databits "Data bits"; stopbit "Stop bit"; remaptxpin "Tx Pin"; remaprxpin "Rx Pin"; flowcontrol "Hardware flow control"; remapctspin "HW Flow control, CTS Pin"; remaprtspin "HW Flow control, RTS Pin"; advanceoptions "Advance options"; rxbuffersize "Rx buffer size (bytes)"; txbuffersize "Tx buffer size (bytes)"; packetmode "Packet mode"; binheader "Binary header (example: '7E 7E')"; binterminator "Binary terminator (example: '03 03')"; porttype_double "Number of data port, type DOUBLE"; porttype_single "Number of data port, type SINGLE"; porttype_int8 "Number of data port, type INT8"; porttype_uint8 "Number of data port, type UINT8"; porttype_int16 "Number of data port, type INT16"; porttype_uint16 "Number of data port, type UINT16"; porttype_int32 "Number of data port, type INT32"; porttype_uint32 "Number of data port, type UINT32"; asciiformat "Ascii format"; rx_asciiterminator "End of packet"; tx_asciiterminator "End of packet"; storagename "Buffer"; varname "Var name"; inputtype "Input data type"; outputtype "Output data type"; binheaderarray "Binary header"; binterminatorarray "Binary terminator"; bindatalength "Binary data length"; asciiheader "Ascii header (printf format)"; asciiterminator "Ascii terminator"; sampletime "Sample time (sec)"; sampletimestr "Compiled sample time (sec) in string"; confstr "Configuration string"; lastmodule "Last module selected"
      mask init:
      | stm32f4_usart_callback('init');
      mask Help: web(fullfile(waijungdocroot,'stm32f4_usart_tx.htm'), '-browser')
      mask TypeOptions configuration: Setup | Tx | Rx
      mask Callback configuration: stm32f4_usart_callback('configuration');
      mask TypeOptions uartmodule: 1 | 2 | 3 | 4 | 5 | 6
      mask Callback uartmodule: stm32f4_usart_callback('uartmodule');
      mask Callback baudrate: stm32f4_usart_callback('baudrate');
      mask TypeOptions databits: 8
      mask TypeOptions parity: No | Odd | Even
      mask TypeOptions stopbit: 0.5 | 1 | 1.5 | 2
      mask TypeOptions remaptxpin: Not used | A9 | B6
      mask TypeOptions remaprxpin: Not used | A10 | B7
      mask TypeOptions flowcontrol: None | RTS | CTS | RTS/CTS
      mask Callback flowcontrol: stm32f4_usart_callback('flowcontrol');
      mask TypeOptions remapctspin: Not used | A11
      mask TypeOptions remaprtspin: Not used | A12
      mask Callback advanceoptions: stm32f4_usart_callback('advanceoptions');
      mask TypeOptions rxbuffersize: 16 | 32 | 64 | 128 | 256 | 512 | 1024 | 2048
      mask TypeOptions txbuffersize: 16 | 32 | 64 | 128 | 256 | 512 | 1024 | 2048
      mask TypeOptions transfer: Blocking | Non-Blocking
      mask Callback transfer: stm32f4_usart_callback('transfer');
      mask TypeOptions packetmode: Ascii | Binary | String Buffer
      mask Callback packetmode: stm32f4_usart_callback('packetmode');
      mask Callback binheader: stm32f4_usart_callback('binheader');
      mask Callback binterminator: stm32f4_usart_callback('binterminator');
      mask Callback porttype_double: stm32f4_usart_callback('porttype');
      mask Callback porttype_single: stm32f4_usart_callback('porttype');
      mask Callback porttype_int8: stm32f4_usart_callback('porttype');
      mask Callback porttype_uint8: stm32f4_usart_callback('porttype');
      mask Callback porttype_int16: stm32f4_usart_callback('porttype');
      mask Callback porttype_uint16: stm32f4_usart_callback('porttype');
      mask Callback porttype_int32: stm32f4_usart_callback('porttype');
      mask Callback porttype_uint32: stm32f4_usart_callback('porttype');
      mask Callback asciiformat: stm32f4_usart_callback('asciiformat');
      mask TypeOptions rx_asciiterminator: CR (0x0D - "\r") | LF (0x0A - "\n") | CRLF (0x0D 0x0A - "\r\n")
      mask Callback rx_asciiterminator: stm32f4_usart_callback('rx_asciiterminator');
      mask TypeOptions tx_asciiterminator: CR (0x0D - "\r") | LF (0x0A - "\n") | CRLF (0x0D 0x0A - "\r\n") | None
      mask Callback tx_asciiterminator: stm32f4_usart_callback('tx_asciiterminator');
      mask TypeOptions storagename: <empty>
      mask Callback storagename: stm32f4_usart_callback('storagename');
      mask Callback varname: stm32f4_usart_callback('varname');
      mask Callback sampletime: stm32f4_usart_callback('sampletime');
      mask Callback sampletimestr: stm32f4_usart_callback('sampletimestr');
      mask Callback blockid: stm32f4_usart_callback('blockid');
      mask Display: text(0.95, 0.5, 'Module: USART2_Tx\nPacket: Binary\nTransfer: Blocking\nTs (sec): -1','ver','middle','hor','right'); port_label('input', 1,'single'); port_label('input', 2,'single'); port_label('input', 3,'single'); port_label('input', 4,'single'); port_label('input', 5,'single'); port_label('input', 6,'single');
  wires:
  UART Rx1/1 -> UART Tx1/6
  UART Rx1/3 -> Terminator1/1
  UART Rx1/5 -> Terminator2/1
  UART Rx1/6 -> Terminator3/1
  UART Rx1/7 -> Terminator4/1
  UART Rx1/8 -> Terminator5/1
  UART Rx1/10 -> Terminator6/1
  UART Rx/1 -> Terminator7/1
  UART Rx/2 -> Terminator8/1
  UART Rx/3 -> Terminator9/1
  UART Rx/4 -> Terminator10/1
  UART Rx/5 -> Terminator11/1
  UART Rx/6 -> Terminator12/1
  UART Rx/9 -> Terminator13/1
  UART Rx1/9 -> UART Tx1/3
  UART Rx1/4 -> UART Tx1/2
  UART Rx1/2 -> UART Tx1/1
  UART Rx/7 -> UART Tx1/4
  UART Rx/8 -> UART Tx1/5
  Logical Operator/1 -> Memory/1, Digital Output/1
  Memory/1 -> Logical Operator/1

== system NE_Red_Rooster_Delta_B_28may/Init_ADXL345 ==
  Enable : EnablePort
  Compare To Zero : simulink/Logic and Bit Operations/Compare To Zero  relop===  OutDataTypeStr=boolean
  Constant : Constant  Value=0
  Constant1 : Constant  Value=hex2dec('A6')  OutDataTypeStr=uint8  SampleTime=-1
  Constant8 : Constant  Value=hex2dec('2D')  OutDataTypeStr=uint8  SampleTime=-1
  Constant9 : Constant  Value=hex2dec('08')  OutDataTypeStr=uint8  SampleTime=-1
  Data Store Write : DataStoreWrite  DataStoreName=Init_ADXL
  Digital Output1 : stm32f4_io_lib/Digital Output  use_bitband=on  port=D  speed=100  porttype=Push Pull  porttypestr=PP  use_pin0=off  use_pin1=off  use_pin2=off  use_pin3=off  use_pin4=off  use_pin5=off  use_pin6=off  use_pin7=off  use_pin8=off  use_pin9=off  use_pin10=off  use_pin11=off  use_pin12=off  use_pin13=on  use_pin14=off  use_pin15=off  pinstr=GPIO_Pin_13  usedpinarray="[0  0  0  0  0  0  0  0  0  0  0  0  0  1  0  0]"  bitbandingstr="#define Init_ADXL345DigitalOutput1_D13 Peripheral_BB(GPIOD->ODR, 13)  /* Output pin */"  sampletime=-1  sampletimestr=-1  blockid=Init_ADXL345DigitalOutput1  enablecustomportlabel=off  globalinit=off  cinputportlabel=In1, In2  coutputportlabel=0
  I2C Master Read/Write1 : stm32f4_i2c_lib/I2C Master Read//Write  configuration=Transaction  module=1  lastmodule=3  transfer=Blocking  dutycycle=TLow/THigh = 2  clkspeed=400  timeout=25  writecount=2  readcount=0  sdapin=C9  sclpin=A8  waitwritetime=0  forcestop=off  inputtypearray=[3 3 3 3]  outputtypearray=[1 3]  confstr="[\"C\",\"9\",\"A\",\"8\",\"1\",\"1\",\"6\",\"0\",\"I2C_DutyCycle_2\",\"0\",\"off\"]"  sampletime=-1  sampletimestr=-1  blockid=Init_ADXL345I2CMasterReadWrite1
  Subsystem : Subsystem
  Terminator : Terminator
  wires:
  Constant9/1 -> I2C Master Read/Write1/3
  I2C Master Read/Write1/1 -> Compare To Zero/1
  Constant1/1 -> I2C Master Read/Write1/1
  Constant8/1 -> I2C Master Read/Write1/2
  Compare To Zero/1 -> Subsystem/Enable
  Subsystem/1(Out1) -> Terminator/1
  Constant/1 -> Digital Output1/1, Data Store Write/1

== system NE_Red_Rooster_Delta_B_28may/Init_L3GD4200  ==
  Enable : EnablePort
  Compare To Zero : simulink/Logic and Bit Operations/Compare To Zero  relop===  OutDataTypeStr=boolean  ZeroCross=off
  Constant : Constant  Value=0
  Data Store Write : DataStoreWrite  DataStoreName=Init_L3GD
  Get Init L3G4200D1 : Subsystem
  Init L3G4200D : Subsystem  TreatAsAtomicUnit=on
  SlvAddr1 : Constant  Value=hex2dec('D2')  OutDataTypeStr=uint8  SampleTime=-1
  wires:
  Compare To Zero/1 -> Init L3G4200D/Enable
  Get Init L3G4200D1/1(Initial Done) -> Compare To Zero/1
  SlvAddr1/1 -> Get Init L3G4200D1/1(SlvAddr)
  Constant/1 -> Data Store Write/1

== system NE_Red_Rooster_Delta_B_28may/Orientation ==
  note: Gyr_X_Roll
  note: Gyr_Y_Pitch
  note: Gyr_Z_Yaw
  Trigger : TriggerPort  VariantControl=Variant
  Accelerometr : Subsystem
  Digital Output1 : stm32f4_io_lib/Digital Output  use_bitband=on  port=D  speed=100  porttype=Push Pull  porttypestr=PP  use_pin0=off  use_pin1=off  use_pin2=off  use_pin3=off  use_pin4=off  use_pin5=off  use_pin6=off  use_pin7=off  use_pin8=off  use_pin9=off  use_pin10=off  use_pin11=off  use_pin12=off  use_pin13=off  use_pin14=on  use_pin15=off  pinstr=GPIO_Pin_14  usedpinarray="[0  0  0  0  0  0  0  0  0  0  0  0  0  0  1  0]"  bitbandingstr="#define OrientationDigitalOutput1_D14 Peripheral_BB(GPIOD->ODR, 14)  /* Output pin */"  sampletime=-1  sampletimestr=-1  blockid=OrientationDigitalOutput1  enablecustomportlabel=off  globalinit=on  cinputportlabel=In1, In2  coutputportlabel=0
  Gyro : Subsystem
  KREN : Subsystem
  KREN_RESULT_ANG : Subsystem
  Logical Operator : Logic  Operator=NOT  AllPortsSameDT=off  OutDataTypeStr=boolean
  Memory : Memory  InheritSampleTime=on
  TANGASCH : Subsystem
  TANGASCH_RESULT_ANG : Subsystem
  Terminator : Terminator
  UART Tx : S-Function  Priority=1  FunctionName=stm32f4_usart  Parameters=configuration,uartmodule,transfer,baudrate,inputtype,outputtype,confstr,binheaderarray,binterminatorarray,asciiheader,asciiterminator,bindatalength,packetmode,varname,sampletime,sampletimestr,blockid  SFunctionDeploymentMode=off  EnableBusSupport=off  mask(stm32f4_usart){configuration=Tx, uartmodule=2, baudrate=115200, databits=8, parity=No, stopbit=1, remaptxpin=Not used, remaprxpin=Not used, flowcontrol=None, remapctspin=Not used, remaprtspin=Not used, advanceoptions=off, rxbuffersize=512, txbuffersize=512, transfer=Blocking, packetmode=Binary, binheader='4F', binterminator='2E', porttype_double=2, porttype_single=0, porttype_int8=0, porttype_uint8=0, porttype_int16=0, porttype_uint16=0, porttype_int32=0, porttype_uint32=0, asciiformat='%1.2f, %1.2f, %1.2f, %1.2f, %1.2f, %1.2f, %i, %i', rx_asciiterminator=CRLF (0x0D 0x0A - "\r\n"), tx_asciiterminator=CRLF (0x0D 0x0A - "\r\n"), storagename=<empty>, varname=, inputtype=[2  0 0], outputtype=[0], binheaderarray=[1 79], binterminatorarray=[1 46], bindatalength=16, asciiheader='%1.2f, %1.2f, %1.2f, %1.2f, %1.2f, %1.2f, %i, %i\r\n', asciiterminator=[2 13 10], sampletime=-1, sampletimestr=-1, blockid=OrientationUARTTx, confstr=[ "dummy", "0", "*", "*", "0", "*", "*", "0", "*", "*", "0", "*", "*", "1", "4", "6", "1", "4", "5", "512", "512", "1", "2", "115200", "8", "No", "1", "None", "USART2"], lastmodule=1}
      mask prompts: uartmodule "UART Module"; baudrate "Baud rate (bps)"; databits "Data bits"; stopbit "Stop bit"; remaptxpin "Tx Pin"; remaprxpin "Rx Pin"; flowcontrol "Hardware flow control"; remapctspin "HW Flow control, CTS Pin"; remaprtspin "HW Flow control, RTS Pin"; advanceoptions "Advance options"; rxbuffersize "Rx buffer size (bytes)"; txbuffersize "Tx buffer size (bytes)"; packetmode "Packet mode"; binheader "Binary header (example: '7E 7E')"; binterminator "Binary terminator (example: '03 03')"; porttype_double "Number of data port, type DOUBLE"; porttype_single "Number of data port, type SINGLE"; porttype_int8 "Number of data port, type INT8"; porttype_uint8 "Number of data port, type UINT8"; porttype_int16 "Number of data port, type INT16"; porttype_uint16 "Number of data port, type UINT16"; porttype_int32 "Number of data port, type INT32"; porttype_uint32 "Number of data port, type UINT32"; asciiformat "Ascii format"; rx_asciiterminator "End of packet"; tx_asciiterminator "End of packet"; storagename "Buffer"; varname "Var name"; inputtype "Input data type"; outputtype "Output data type"; binheaderarray "Binary header"; binterminatorarray "Binary terminator"; bindatalength "Binary data length"; asciiheader "Ascii header (printf format)"; asciiterminator "Ascii terminator"; sampletime "Sample time (sec)"; sampletimestr "Compiled sample time (sec) in string"; confstr "Configuration string"; lastmodule "Last module selected"
      mask help:
      | Data type for Ascii format
      | %u, %i, %d, %o, %x: uint32
      | %e, %g, %f: single
      | %c: int8
      mask init:
      | stm32f4_usart_callback('init');
      mask Help: web(fullfile(waijungdocroot,'stm32f4_usart_tx.htm'), '-browser')
      mask TypeOptions configuration: Setup | Tx | Rx
      mask Callback configuration: stm32f4_usart_callback('configuration');
      mask TypeOptions uartmodule: 1 | 2 | 3 | 4 | 5 | 6
      mask Callback uartmodule: stm32f4_usart_callback('uartmodule');
      mask Callback baudrate: stm32f4_usart_callback('baudrate');
      mask TypeOptions databits: 8
      mask TypeOptions parity: No | Odd | Even
      mask TypeOptions stopbit: 0.5 | 1 | 1.5 | 2
      mask TypeOptions remaptxpin: Not used | A9 | B6
      mask TypeOptions remaprxpin: Not used | A10 | B7
      mask TypeOptions flowcontrol: None | RTS | CTS | RTS/CTS
      mask Callback flowcontrol: stm32f4_usart_callback('flowcontrol');
      mask TypeOptions remapctspin: Not used | A11
      mask TypeOptions remaprtspin: Not used | A12
      mask Callback advanceoptions: stm32f4_usart_callback('advanceoptions');
      mask TypeOptions rxbuffersize: 16 | 32 | 64 | 128 | 256 | 512 | 1024 | 2048
      mask TypeOptions txbuffersize: 16 | 32 | 64 | 128 | 256 | 512 | 1024 | 2048
      mask TypeOptions transfer: Blocking | Non-Blocking
      mask Callback transfer: stm32f4_usart_callback('transfer');
      mask TypeOptions packetmode: Ascii | Binary | Binary Vector | String Buffer | Raw Buffer
      mask Callback packetmode: stm32f4_usart_callback('packetmode');
      mask Callback binheader: stm32f4_usart_callback('binheader');
      mask Callback binterminator: stm32f4_usart_callback('binterminator');
      mask Callback porttype_double: stm32f4_usart_callback('porttype');
      mask Callback porttype_single: stm32f4_usart_callback('porttype');
      mask Callback porttype_int8: stm32f4_usart_callback('porttype');
      mask Callback porttype_uint8: stm32f4_usart_callback('porttype');
      mask Callback porttype_int16: stm32f4_usart_callback('porttype');
      mask Callback porttype_uint16: stm32f4_usart_callback('porttype');
      mask Callback porttype_int32: stm32f4_usart_callback('porttype');
      mask Callback porttype_uint32: stm32f4_usart_callback('porttype');
      mask Callback asciiformat: stm32f4_usart_callback('asciiformat');
      mask TypeOptions rx_asciiterminator: CR (0x0D - "\r") | LF (0x0A - "\n") | CRLF (0x0D 0x0A - "\r\n")
      mask Callback rx_asciiterminator: stm32f4_usart_callback('rx_asciiterminator');
      mask TypeOptions tx_asciiterminator: CR (0x0D - "\r") | LF (0x0A - "\n") | CRLF (0x0D 0x0A - "\r\n") | None
      mask Callback tx_asciiterminator: stm32f4_usart_callback('tx_asciiterminator');
      mask TypeOptions storagename: <empty>
      mask Callback storagename: stm32f4_usart_callback('storagename');
      mask Callback varname: stm32f4_usart_callback('varname');
      mask Callback sampletime: stm32f4_usart_callback('sampletime');
      mask Callback sampletimestr: stm32f4_usart_callback('sampletimestr');
      mask Callback blockid: stm32f4_usart_callback('blockid');
      mask Display: text(0.95, 0.5, 'Module: USART2_Tx\nPacket: Binary\nTransfer: Blocking\nTs (sec): -1','ver','middle','hor','right'); port_label('input', 1,'double'); port_label('input', 2,'double');
  wires:
  Gyro/1(Out1) -> Terminator/1
  Accelerometr/1(Axe_X) -> TANGASCH/3(Xa_F), KREN/2(Xa_F)
  Accelerometr/2(Axe_Y) -> KREN/3(Ya_F), TANGASCH/2(Ya_F)
  Accelerometr/3(Axe_Z) -> KREN/1(Za_F), TANGASCH/1(Za_F)
  Gyro/3(Out3) -> TANGASCH_RESULT_ANG/1(Gyr_Data)
  Gyro/2(Out2) -> KREN_RESULT_ANG/1(Gyr_Data)
  TANGASCH/1(ACC_Pitch) -> KREN_RESULT_ANG/2(Acc_Data)
  KREN/1(ACC_Roll) -> TANGASCH_RESULT_ANG/2(Acc_Data)
  KREN_RESULT_ANG/1(Out1) -> UART Tx/1
  TANGASCH_RESULT_ANG/1(Out1) -> UART Tx/2
  Logical Operator/1 -> Digital Output1/1, Memory/1
  Memory/1 -> Logical Operator/1

== system NE_Red_Rooster_Delta_B_28may/Reset_Subsystem ==
  Compare To Constant : simulink/Logic and Bit Operations/Compare To Constant  relop===  const=1.0  OutDataTypeStr=boolean
  Digital Input : stm32f4_io_lib/Digital Input  port=A  speed=100  porttype=None  porttypestr=NOPULL  use_pin0=on  use_pin1=off  use_pin2=off  use_pin3=off  use_pin4=off  use_pin5=off  use_pin6=off  use_pin7=off  use_pin8=off  use_pin9=off  use_pin10=off  use_pin11=off  use_pin12=off  use_pin13=off  use_pin14=off  use_pin15=off  pinstr=GPIO_Pin_0  usedpinarray="[1  0  0  0  0  0  0  0  0  0  0  0  0  0  0  0]"  bitbandingstr="#define Reset_SubsystemDigitalInput_A0 Peripheral_BB(GPIOA->IDR, 0)  /* Output pin */"  sampletime=-1  sampletimestr=0.0005  blockid=Reset_SubsystemDigitalInput  enablecustomportlabel=off  glabalinit=off  cinputportlabel=In1, In2  coutputportlabel=Out1, Out2
  Enabled Subsystem : Subsystem  TreatAsAtomicUnit=on
  wires:
  Compare To Constant/1 -> Enabled Subsystem/Enable
  Digital Input/1 -> Compare To Constant/1
